simulink model "current_inverter"  (R2023a)
settings: Solver=ode4  StartTime=0.0  StopTime=0.8  FixedStep=1e-6  RelTol=1e-3
undefined symbols (not defined in the file): omega, vref_rms
libraries: spsThreePhaseVIMeasurementLib x5, spsHalfBridgeConverterLib x3, spsGroundLib x2, eeGeneralControl x2, spsPower3phInstantaneousLib x2, spsThreePhaseSeriesRLCBranchLib x2, spsAlphaBetaZerotoabcLib x1, spsDCVoltageSourceLib x1, spsPLL3phLib x1, spsRMSLib x1, eePwmGeneratorTwoLevel x1, spsThreePhaseParallelRLCBranchLib x1
settings Model: Creator=MrSam  LastModifiedBy=15185

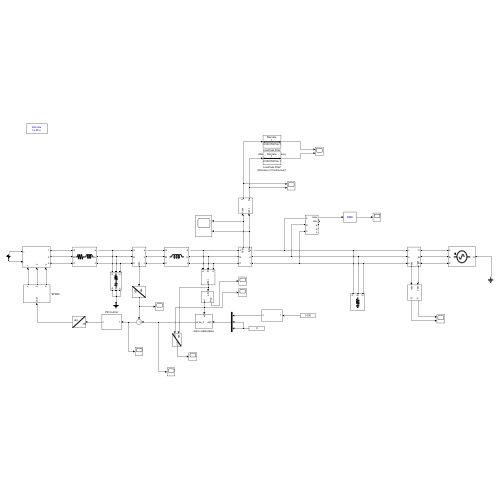
[thumbnail: Simulink's stored preview of the top-level diagram]
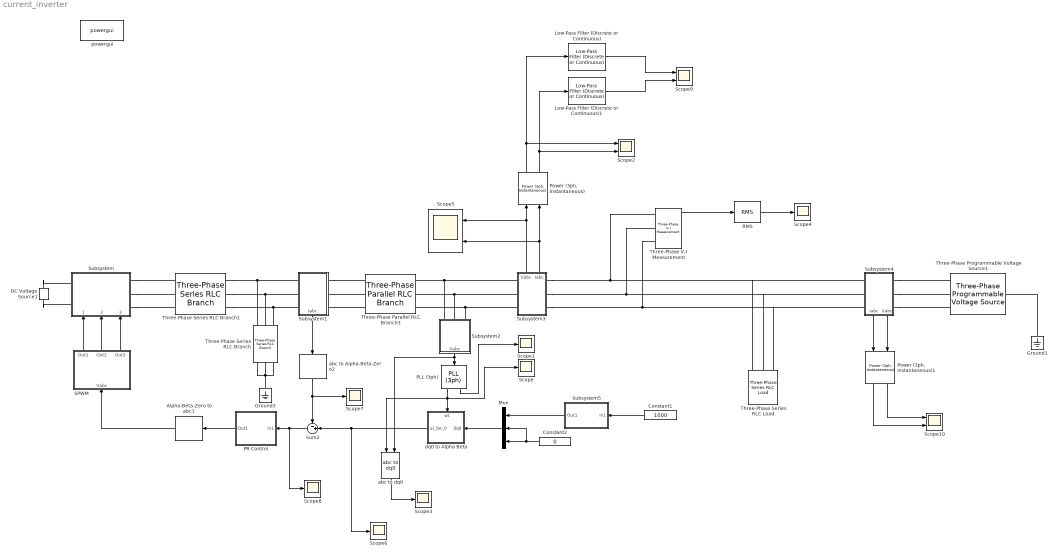
== system current_inverter ==
  Alpha-Beta-Zero to abc1 : spsAlphaBetaZerotoabcLib/Alpha-Beta-Zero to abc
      settings: LibrarySourceBlock=|
      | sps_lib/Control/Alpha-Beta-Zero
      | to abc
  Constant1 : Constant  Value=1000
  Constant2 : Constant  Value=0
  DC Voltage Source1 : spsDCVoltageSourceLib/DC Voltage Source  Amplitude=600  Measurements=None
  Ground1 : spsGroundLib/Ground  LConnTagsString=a
  Ground3 : spsGroundLib/Ground  LConnTagsString=a
  Low-Pass Filter (Discrete or Continuous) : eeGeneralControl/Low-Pass Filter (Discrete or Continuous)  K=1  T=1/(2*pi*1000)  B=inf  A=-inf  init_option=Inherited from block input  x0=0  Ts=-1
  Low-Pass Filter (Discrete or Continuous)1 : eeGeneralControl/Low-Pass Filter (Discrete or Continuous)  K=1  T=1/(2*pi*1000)  B=inf  A=-inf  init_option=Inherited from block input  x0=0  Ts=-1
  Mux : Mux  Inputs=3
  PLL (3ph) : spsPLL3phLib/PLL (3ph)  Fmin=45  Par_Init=[0, 50]  ParK=[180, 3200, 1]  TcD=1e-4  MaxRateChangeFreq=12  FilterCutOffFreq=25  Ts=0  AGC=on
  PR Control : Subsystem
  "Power (3ph, Instantaneous)" : spsPower3phInstantaneousLib/Power (3ph, Instantaneous)
  "Power (3ph, Instantaneous)1" : spsPower3phInstantaneousLib/Power (3ph, Instantaneous)
  RMS : spsRMSLib/RMS  TrueRMS=on  Freq=50  RMSInit=120  Ts=0
  SPWM : Subsystem
  Scope{,1,3..4,6..8} (7 alike) : Scope
  Scope{2,5,9..10} (4 alike) : Scope  NumInputPorts=2
  Subsystem : Subsystem
      settings: PortSchema="{\"entries\":[{\"content\":{\"sides\":[{\"content\":{\"connectorIds\":[\"LConn1\",\"LConn2\"]},\"type\":\"ConnectorPlacement.EquallySpacedRectSide\",\"uuid\":\"21765539-0567-4900-b052-fb0c809e49e6\"},{\"content\":{\"connectorIds\":[\"RConn1\",\"RConn2\",\"RConn3\"],\"side\":\"RIGHT\"},\"type\":\"ConnectorPlacement.EquallySpacedRectSide\",\"uuid\":\"da60e673-aefd-4ef6-b5b1-e42a137712f7\"},{\"content\":{\"side\":\"TOP\"},\"type\":\"ConnectorPlacement.EquallySpacedRectSide\",\"uuid\":\"b6e664be-1a8c-4c9c-bd73-b93bd6e53381\"},{\"content\":{\"connectorIds\":[\"In1\",\"In2\",\"In3\"],\"side\":\"BOTTOM\"},\"type\":\"ConnectorPlacement.EquallySpacedRectSide\",\"uuid\":\"f785bed7-33ce-41e0-9620-ddd9724794f7\"}]},\"type\":\"ConnectorPlacement.EquallySpacedConnector\",\"uuid\":\"3eaff965-cae1-44ee-8f3f-ae8df46f200b\"}],\"packageUris\":[\"http://schema.mathworks.com/mf0/Connector/R2020b\"],\"version\":\"1.0\"}"
  Subsystem1 : Subsystem
      settings: PortSchema="{\"entries\":[{\"content\":{\"sides\":[{\"content\":{\"connectorIds\":[\"LConn1\",\"LConn2\",\"LConn3\"]},\"type\":\"ConnectorPlacement.EquallySpacedRectSide\",\"uuid\":\"5e649b81-8d67-47fb-b51d-7fa1d294a0fa\"},{\"content\":{\"connectorIds\":[\"RConn1\",\"RConn2\",\"RConn3\"],\"side\":\"RIGHT\"},\"type\":\"ConnectorPlacement.EquallySpacedRectSide\",\"uuid\":\"b8ce6232-1e24-4620-bb1d-7a04b9b53c9d\"},{\"content\":{\"side\":\"TOP\"},\"type\":\"ConnectorPlacement.EquallySpacedRectSide\",\"uuid\":\"aabe5581-fbc6-4714-8701-49215a0525de\"},{\"content\":{\"connectorIds\":[\"Out1\"],\"side\":\"BOTTOM\"},\"type\":\"ConnectorPlacement.EquallySpacedRectSide\",\"uuid\":\"d004e6ed-4fae-491a-82a2-0495bcb0f8c1\"}]},\"type\":\"ConnectorPlacement.EquallySpacedConnector\",\"uuid\":\"9c494b08-2ee2-4375-b64d-9899f5cce3ba\"}],\"packageUris\":[\"http://schema.mathworks.com/mf0/Connector/R2020b\"],\"version\":\"1.0\"}"
  Subsystem2 : Subsystem
  Subsystem3 : Subsystem
      settings: PortSchema="{\"entries\":[{\"content\":{\"sides\":[{\"content\":{\"connectorIds\":[\"LConn1\",\"LConn2\",\"LConn3\"]},\"type\":\"ConnectorPlacement.EquallySpacedRectSide\",\"uuid\":\"5e649b81-8d67-47fb-b51d-7fa1d294a0fa\"},{\"content\":{\"connectorIds\":[\"RConn1\",\"RConn2\",\"RConn3\"],\"side\":\"RIGHT\"},\"type\":\"ConnectorPlacement.EquallySpacedRectSide\",\"uuid\":\"b8ce6232-1e24-4620-bb1d-7a04b9b53c9d\"},{\"content\":{\"connectorIds\":[\"Out1\",\"Out2\"],\"side\":\"TOP\"},\"type\":\"ConnectorPlacement.EquallySpacedRectSide\",\"uuid\":\"aabe5581-fbc6-4714-8701-49215a0525de\"}]},\"type\":\"ConnectorPlacement.EquallySpacedConnector\",\"uuid\":\"9c494b08-2ee2-4375-b64d-9899f5cce3ba\"}],\"packageUris\":[\"http://schema.mathworks.com/mf0/Connector/R2020b\"],\"version\":\"1.0\"}"
  Subsystem4 : Subsystem
      settings: PortSchema="{\"entries\":[{\"content\":{\"sides\":[{\"content\":{\"connectorIds\":[\"LConn1\",\"LConn2\",\"LConn3\"]},\"type\":\"ConnectorPlacement.EquallySpacedRectSide\",\"uuid\":\"5e649b81-8d67-47fb-b51d-7fa1d294a0fa\"},{\"content\":{\"connectorIds\":[\"RConn1\",\"RConn2\",\"RConn3\"],\"side\":\"RIGHT\"},\"type\":\"ConnectorPlacement.EquallySpacedRectSide\",\"uuid\":\"b8ce6232-1e24-4620-bb1d-7a04b9b53c9d\"},{\"content\":{\"connectorIds\":[\"Out1\",\"Out2\"],\"side\":\"TOP\"},\"type\":\"ConnectorPlacement.EquallySpacedRectSide\",\"uuid\":\"aabe5581-fbc6-4714-8701-49215a0525de\"}]},\"type\":\"ConnectorPlacement.EquallySpacedConnector\",\"uuid\":\"9c494b08-2ee2-4375-b64d-9899f5cce3ba\"}],\"packageUris\":[\"http://schema.mathworks.com/mf0/Connector/R2020b\"],\"version\":\"1.0\"}"
  Subsystem5 : Subsystem
  Sum2 : Sum  Inputs=-+|
  Three-Phase Parallel RLC Branch3 : spsThreePhaseParallelRLCBranchLib/Three-Phase Parallel RLC Branch  LConnTagsString=A|B|C  RConnTagsString=A|B|C  BranchType=L  Resistance=1  Inductance=0.00024  Capacitance=1e-6  Measurements=None
  Three-Phase Programmable Voltage Source1 : spsThreePhaseProgrammableVoltageSourceLib/Three-Phase Programmable Voltage Source  PositiveSequence="[vref_rms  0 50]"  VariationEntity=None  VariationType=Table of time-amplitude pairs  VariationTypeAlt=Step  VariationStep=0.5  VariationRate=10  VariationMagnitude=0.3  VariationFrequency=2  VariationTiming=[1 2]  VariationPhaseA=off  Amplitudes=[1 0.8 1.2 1.0]  TimeValues=[0 0.1 0.15 0.2]  HarmonicGeneration=off  HarmonicA=[3 0.2 -25 0]  HarmonicB=[2 0.15 35 2]  Timing="[0.05  3]"  BusType=swing  Pref=0  Qref=0  Qmin=-inf  Qmax=inf
  Three-Phase Series RLC Branch : spsThreePhaseSeriesRLCBranchLib/Three-Phase Series RLC Branch  LConnTagsString=A|B|C  RConnTagsString=A|B|C  BranchType=RC  Resistance=1  Inductance=1e-3  Capacitance=2e-05  Measurements=None
  Three-Phase Series RLC Branch1 : spsThreePhaseSeriesRLCBranchLib/Three-Phase Series RLC Branch  LConnTagsString=A|B|C  RConnTagsString=A|B|C  BranchType=RL  Resistance=0.3  Inductance=0.004  Capacitance=1e-6  Measurements=None
  Three-Phase Series RLC Load : spsThreePhaseSeriesRLCLoadLib/Three-Phase Series RLC Load  LConnTagsString=A|B|C  Configuration=Y (grounded)  NominalVoltage=367  Vabc=[1e3 1e3 1e3]  Vabcp=[1e3 1e3 1e3]  NominalFrequency=50  UnbalancedPower=off  ActivePower=1000  InductivePower=0  CapacitivePower=0  Pabc=[10e3 9e3 11e3]  QLabc=[100 90 110]  QCabc=[100 90 110]  Pabcp=[10e3 9e3 11e3]  QLabcp=[100 90 110]  QCabcp=[100 90 110]  Measurements=None  LoadType=constant Z
  Three-Phase V-I Measurement : spsThreePhaseVIMeasurementLib/Three-Phase V-I Measurement  VoltageMeasurement=phase-to-phase  SetLabelV=off  LabelV=Vabc  Vpu=off  VpuLL=off  CurrentMeasurement=yes  SetLabelI=off  LabelI=Iabc  Ipu=off  Pbase=100e6  Vbase=500e3  OutputType=Complex  PhasorSimulation=off  PSBequivalent=0
  abc to Alpha-Beta-Zero2 : spsabctoAlphaBetaZeroLib/abc to Alpha-Beta-Zero
  abc to dq0 : spsabctodq0Lib/abc to dq0  Alignment=90 degrees behind phase A axis
  dq0 to Alpha Beta : Subsystem
      settings: PortSchema="{\"entries\":[{\"content\":{\"sides\":[{\"content\":{\"connectorIds\":[\"In1\"]},\"type\":\"ConnectorPlacement.EquallySpacedRectSide\",\"uuid\":\"2957cf7a-c1c3-4848-9407-b6952c647f30\"},{\"content\":{\"connectorIds\":[\"Out1\"],\"side\":\"RIGHT\"},\"type\":\"ConnectorPlacement.EquallySpacedRectSide\",\"uuid\":\"7a8beffb-254d-479d-a697-96ba44ae1442\"},{\"content\":{\"connectorIds\":[\"In2\"],\"side\":\"TOP\"},\"type\":\"ConnectorPlacement.EquallySpacedRectSide\",\"uuid\":\"8b95608f-2c8d-45bf-9e71-a12dce74a0a0\"}]},\"type\":\"ConnectorPlacement.EquallySpacedConnector\",\"uuid\":\"69f38502-e33d-4dbf-872c-0372c4b36551\"}],\"packageUris\":[\"http://schema.mathworks.com/mf0/Connector/R2020b\"],\"version\":\"1.0\"}"
  powergui : spspowerguiLib/powergui  Priority=1  SimulationMode=Discrete  SampleTime=1e-6  frequency=60  Iterations=50  frequencyindice=50  Pbase=100e6  ErrMax=1e-4  UnitsV=kV  UnitsW=MW  buscounter=0  FunctionMessages=off  echomessages=off  EnableUseOfTLC=off  CurrentSourceSwitches=off  DisableSnubberDevices=off  DisableRonSwitches=off  DisableVfSwitches=off  DisplayEquations=off  AutomaticDiscreteSolvers=off  SolverType=Tustin/Backward Euler (TBE)  Interpol=off  ExternalGateDelay=off  methode=off  Ts=100  x0status=blocks  SPID=on  SwTol=0  HookPort=off  NonlinearTolerance=1e-4  nMaxIteration=100  ContinueOnMaxIteration=off  RestoreLinks=warning  ResistiveCurrentMeasurement=off  Frange=[0:2:500]  Ylog=off  Xlog=on  ShowGrid=off  save=off  variable=ZData  structure=0  ZoomFFT=off  StartTime=0.0  cycles=1  DisplayStyle=1  fundamental=60  FreqAxis=off  MaxFrequency=1000  frequencyindicesteady=1  RmsSteady=1  display=off
  wires:
  SPWM/1(Out1) -> Subsystem/1(" 1 ")
  SPWM/2(Out2) -> Subsystem/2("  2")
  SPWM/3(Out3) -> Subsystem/3("  3")
  Subsystem1/1(Iabc) -> abc to Alpha-Beta-Zero2/1
  Subsystem3/2(Iabc) -> Scope5/2, "Power (3ph, Instantaneous)"/2
  Subsystem3/1(Vabc) -> "Power (3ph, Instantaneous)"/1, Scope5/1
  Sum2/1 -> Scope8/1, PR Control/1(In1)
  PR Control/1(Out1) -> Alpha-Beta-Zero to abc1/1
  Subsystem2/1(Vabc) -> abc to dq0/1, PLL (3ph)/1
  dq0 to Alpha Beta/1(al_be_0) -> Scope6/1, Sum2/2
  Mux/1 -> dq0 to Alpha Beta/1(dq0)
  PLL (3ph)/2 -> abc to dq0/2, dq0 to Alpha Beta/2(wt), Scope/1
  Constant2/1 -> Mux/2, Mux/3
  PLL (3ph)/1 -> Scope1/1
  "Power (3ph, Instantaneous)"/1 -> Low-Pass Filter (Discrete or Continuous)/1, Scope2/1
  "Power (3ph, Instantaneous)"/2 -> Low-Pass Filter (Discrete or Continuous)1/1, Scope2/2
  abc to dq0/1 -> Scope3/1
  Alpha-Beta-Zero to abc1/1 -> SPWM/1(Vabc)
  abc to Alpha-Beta-Zero2/1 -> Scope7/1, Sum2/1
  Low-Pass Filter (Discrete or Continuous)/1 -> Scope9/1
  Low-Pass Filter (Discrete or Continuous)1/1 -> Scope9/2
  Three-Phase V-I Measurement/1 -> RMS/1
  RMS/1 -> Scope4/1
  Subsystem4/2(Iabc) -> "Power (3ph, Instantaneous)1"/2
  Subsystem4/1(Vabc) -> "Power (3ph, Instantaneous)1"/1
  "Power (3ph, Instantaneous)1"/1 -> Scope10/1
  "Power (3ph, Instantaneous)1"/2 -> Scope10/2
  Subsystem5/1(Out1) -> Mux/1
  Constant1/1 -> Subsystem5/1(In1)
  connections:
  Ground3/LConn1 -- Three-Phase Series RLC Branch/RConn3 -- Three-Phase Series RLC Branch/RConn1 -- Three-Phase Series RLC Branch/RConn2
  DC Voltage Source1/RConn1 -- Subsystem/LConn1
  DC Voltage Source1/LConn1 -- Subsystem/LConn2
  Three-Phase Series RLC Branch/LConn1 -- Three-Phase Series RLC Branch1/RConn1 -- Subsystem1/LConn1
  Three-Phase Series RLC Branch/LConn2 -- Three-Phase Series RLC Branch1/RConn2 -- Subsystem1/LConn2
  Three-Phase Series RLC Branch/LConn3 -- Three-Phase Series RLC Branch1/RConn3 -- Subsystem1/LConn3
  Subsystem1/RConn1 -- Three-Phase Parallel RLC Branch3/LConn1
  Subsystem1/RConn2 -- Three-Phase Parallel RLC Branch3/LConn2
  Subsystem1/RConn3 -- Three-Phase Parallel RLC Branch3/LConn3
  Subsystem2/LConn1 -- Three-Phase Parallel RLC Branch3/RConn1 -- Subsystem3/LConn1
  Subsystem2/LConn2 -- Three-Phase Parallel RLC Branch3/RConn2 -- Subsystem3/LConn2
  Subsystem2/LConn3 -- Three-Phase Parallel RLC Branch3/RConn3 -- Subsystem3/LConn3
  Subsystem3/RConn1 -- Subsystem4/RConn3 -- Three-Phase Series RLC Load/LConn1 -- Three-Phase V-I Measurement/LConn1
  Subsystem3/RConn2 -- Subsystem4/RConn2 -- Three-Phase Series RLC Load/LConn2 -- Three-Phase V-I Measurement/LConn2
  Subsystem3/RConn3 -- Subsystem4/RConn1 -- Three-Phase Series RLC Load/LConn3 -- Three-Phase V-I Measurement/LConn3
  Ground1/LConn1 -- Three-Phase Programmable Voltage Source1/LConn1
  Subsystem/RConn2 -- Three-Phase Series RLC Branch1/LConn2
  Subsystem/RConn1 -- Three-Phase Series RLC Branch1/LConn1
  Subsystem/RConn3 -- Three-Phase Series RLC Branch1/LConn3
  Subsystem4/LConn3 -- Three-Phase Programmable Voltage Source1/RConn1
  Subsystem4/LConn2 -- Three-Phase Programmable Voltage Source1/RConn2
  Subsystem4/LConn1 -- Three-Phase Programmable Voltage Source1/RConn3

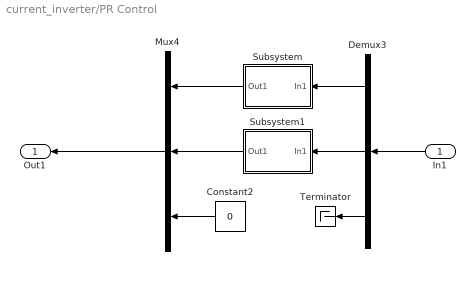
== system current_inverter/PR Control ==
  In1 : Inport
  Constant2 : Constant  Value=0
  Demux3 : Demux  Outputs=3
  Mux4 : Mux  Inputs=3
  Subsystem : Subsystem
  Subsystem1 : Subsystem
  Terminator : Terminator
  Out1 : Outport
  wires:
  Mux4/1 -> Out1/1
  Constant2/1 -> Mux4/3
  In1/1 -> Demux3/1
  Demux3/3 -> Terminator/1
  Demux3/1 -> Subsystem/1(In1)
  Subsystem/1(Out1) -> Mux4/1
  Subsystem1/1(Out1) -> Mux4/2
  Demux3/2 -> Subsystem1/1(In1)

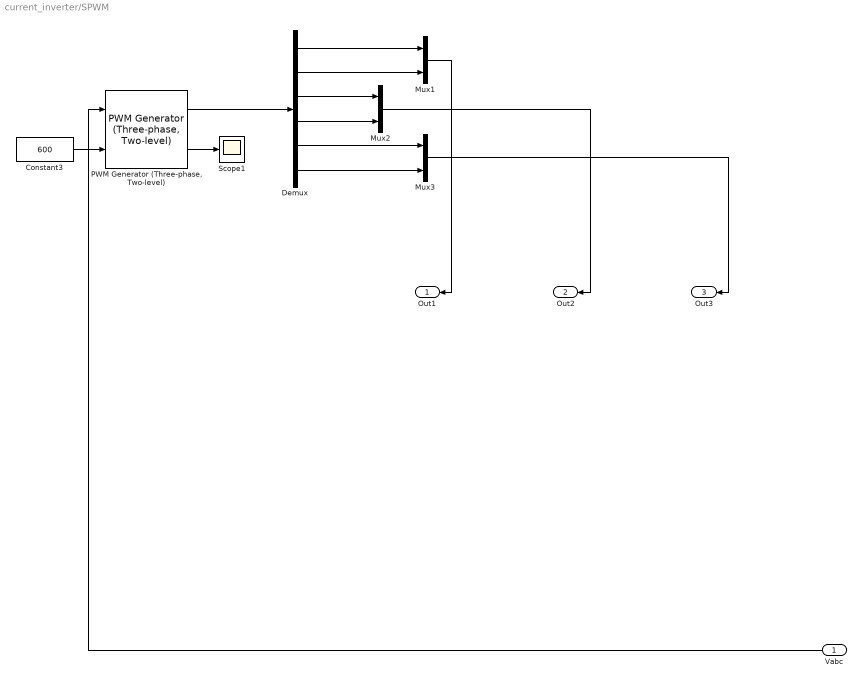
== system current_inverter/SPWM ==
  Vabc : Inport
  Constant3 : Constant  Value=600
  Demux : Demux  Outputs=6
  Mux1 : Mux  Inputs=2
  Mux2 : Mux  Inputs=2
  Mux3 : Mux  Inputs=2
  "PWM Generator (Three-phase, Two-level)" : eePwmGeneratorTwoLevel/PWM Generator (Three-phase, Two-level)  PWMMode=Continuous PWM (CPWM)  CPWMMode=SPWM: sinusoidal PWM  DPWMMode=60 DPWM: 60 degree discontinuous PWM  fsw=10000  Ts=1/(100*10000)
      settings: LibrarySourceBlock=|
      | ee_sl_lib/Pulse Width
      | Modulation/PWM Generator
      | (Three-phase, Two-level)
  Scope1 : Scope
  Out1 : Outport
  Out2 : Outport  Port=2
  Out3 : Outport  Port=3
  wires:
  "PWM Generator (Three-phase, Two-level)"/2 -> Scope1/1
  Demux/2 -> Mux1/2
  Vabc/1 -> "PWM Generator (Three-phase, Two-level)"/1
  Demux/6 -> Mux3/2
  Demux/1 -> Mux1/1
  Constant3/1 -> "PWM Generator (Three-phase, Two-level)"/2
  Mux2/1 -> Out2/1
  Demux/4 -> Mux2/2
  "PWM Generator (Three-phase, Two-level)"/1 -> Demux/1
  Demux/3 -> Mux2/1
  Demux/5 -> Mux3/1
  Mux1/1 -> Out1/1
  Mux3/1 -> Out3/1

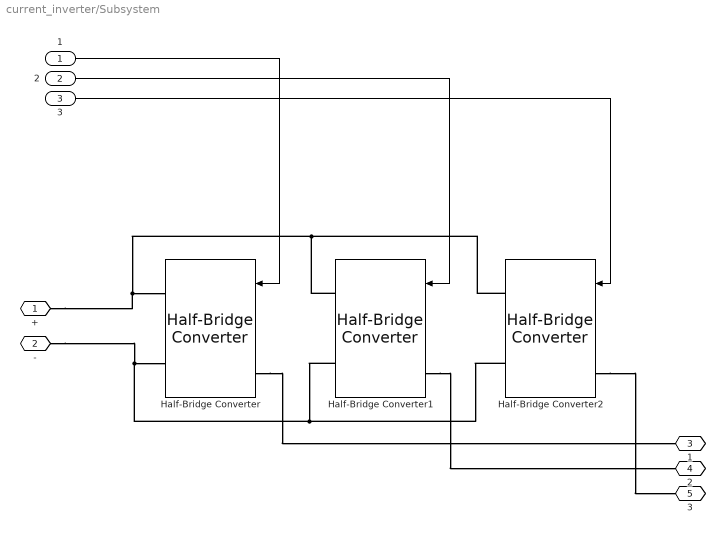
== system current_inverter/Subsystem ==
  " 1 " : Inport
  "  2" : Inport  Port=2
  "  3" : Inport  Port=3
  Half-Bridge Converter : spsHalfBridgeConverterLib/Half-Bridge Converter  ModelType=Switching devices  Ron=1e-3  Rs=1e6  Cs=inf  Vforward=[0,0]  Ron_Diode=1e-3  Rs_Diode=1e6  Cs_Diode=inf  Vf_Diode=1e-3  Rs_CurrentSource=inf  Ron_ACsource=1e-3
      settings: LibrarySourceBlock=sps_lib/Power Electronics/Half-Bridge Converter
  Half-Bridge Converter1 : spsHalfBridgeConverterLib/Half-Bridge Converter  ModelType=Switching devices  Ron=1e-3  Rs=1e6  Cs=inf  Vforward=[0,0]  Ron_Diode=1e-3  Rs_Diode=1e6  Cs_Diode=inf  Vf_Diode=1e-3  Rs_CurrentSource=inf  Ron_ACsource=1e-3
      settings: LibrarySourceBlock=sps_lib/Power Electronics/Half-Bridge Converter
  Half-Bridge Converter2 : spsHalfBridgeConverterLib/Half-Bridge Converter  ModelType=Switching devices  Ron=1e-3  Rs=1e6  Cs=inf  Vforward=[0,0]  Ron_Diode=1e-3  Rs_Diode=1e6  Cs_Diode=inf  Vf_Diode=1e-3  Rs_CurrentSource=inf  Ron_ACsource=1e-3
      settings: LibrarySourceBlock=sps_lib/Power Electronics/Half-Bridge Converter
  + : PMIOPort  Side=Left
  - : PMIOPort  Port=2  Side=Left
  1 : PMIOPort  Port=3  Side=Right
  2 : PMIOPort  Port=4  Side=Right
  3 : PMIOPort  Port=5  Side=Right
  wires:
  "  2"/1 -> Half-Bridge Converter1/1
  "  3"/1 -> Half-Bridge Converter2/1
  " 1 "/1 -> Half-Bridge Converter/1
  connections:
  Half-Bridge Converter/LConn1 -- 1/RConn1
  Half-Bridge Converter2/RConn1 -- Half-Bridge Converter1/RConn1 -- Half-Bridge Converter/RConn1 -- +/RConn1
  Half-Bridge Converter2/RConn2 -- Half-Bridge Converter1/RConn2 -- Half-Bridge Converter/RConn2 -- -/RConn1
  Half-Bridge Converter2/LConn1 -- 3/RConn1
  Half-Bridge Converter1/LConn1 -- 2/RConn1

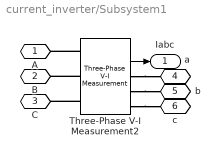
== system current_inverter/Subsystem1 ==
  Three-Phase V-I Measurement2 : spsThreePhaseVIMeasurementLib/Three-Phase V-I Measurement  VoltageMeasurement=phase-to-ground  SetLabelV=off  LabelV=Vabc  Vpu=off  VpuLL=off  CurrentMeasurement=yes  SetLabelI=off  LabelI=Iabc  Ipu=off  Pbase=100e6  Vbase=500e3  OutputType=Complex  PhasorSimulation=off  PSBequivalent=0
  A : PMIOPort  Side=Left
  B : PMIOPort  Port=2  Side=Left
  C : PMIOPort  Port=3  Side=Left
  a : PMIOPort  Port=4  Side=Right
  b : PMIOPort  Port=5  Side=Right
  c : PMIOPort  Port=6  Side=Right
  Iabc : Outport
  wires:
  Three-Phase V-I Measurement2/2 -> Iabc/1
  connections:
  Three-Phase V-I Measurement2/LConn1 -- A/RConn1
  Three-Phase V-I Measurement2/RConn3 -- c/RConn1
  Three-Phase V-I Measurement2/RConn1 -- a/RConn1
  Three-Phase V-I Measurement2/LConn2 -- B/RConn1
  Three-Phase V-I Measurement2/RConn2 -- b/RConn1
  Three-Phase V-I Measurement2/LConn3 -- C/RConn1

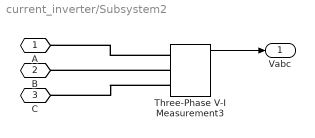
== system current_inverter/Subsystem2 ==
  Three-Phase V-I Measurement3 : spsThreePhaseVIMeasurementLib/Three-Phase V-I Measurement  VoltageMeasurement=phase-to-ground  SetLabelV=off  LabelV=Vabc  Vpu=off  VpuLL=off  CurrentMeasurement=yes  SetLabelI=off  LabelI=Iabc  Ipu=off  Pbase=100e6  Vbase=500e3  OutputType=Complex  PhasorSimulation=off  PSBequivalent=0
  A : PMIOPort  Side=Left
  B : PMIOPort  Port=2  Side=Left
  C : PMIOPort  Port=3  Side=Left
  Vabc : Outport
  wires:
  Three-Phase V-I Measurement3/1 -> Vabc/1
  connections:
  Three-Phase V-I Measurement3/LConn1 -- A/RConn1
  Three-Phase V-I Measurement3/LConn2 -- B/RConn1
  Three-Phase V-I Measurement3/LConn3 -- C/RConn1

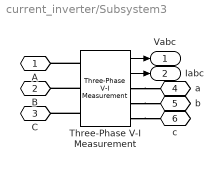
== system current_inverter/Subsystem3 ==
  Three-Phase V-I Measurement : spsThreePhaseVIMeasurementLib/Three-Phase V-I Measurement  VoltageMeasurement=phase-to-ground  SetLabelV=off  LabelV=Vabc  Vpu=off  VpuLL=off  CurrentMeasurement=yes  SetLabelI=off  LabelI=Iabc  Ipu=off  Pbase=100e6  Vbase=500e3  OutputType=Complex  PhasorSimulation=off  PSBequivalent=0
  A : PMIOPort  Side=Left
  B : PMIOPort  Port=2  Side=Left
  C : PMIOPort  Port=3  Side=Left
  a : PMIOPort  Port=4  Side=Right
  b : PMIOPort  Port=5  Side=Right
  c : PMIOPort  Port=6  Side=Right
  Vabc : Outport
  Iabc : Outport  Port=2
  wires:
  Three-Phase V-I Measurement/2 -> Iabc/1
  Three-Phase V-I Measurement/1 -> Vabc/1
  connections:
  Three-Phase V-I Measurement/RConn1 -- a/RConn1
  Three-Phase V-I Measurement/LConn2 -- B/RConn1
  Three-Phase V-I Measurement/RConn3 -- c/RConn1
  Three-Phase V-I Measurement/LConn1 -- A/RConn1
  Three-Phase V-I Measurement/LConn3 -- C/RConn1
  Three-Phase V-I Measurement/RConn2 -- b/RConn1

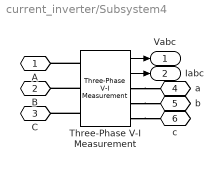
== system current_inverter/Subsystem4 ==
  Three-Phase V-I Measurement : spsThreePhaseVIMeasurementLib/Three-Phase V-I Measurement  VoltageMeasurement=phase-to-ground  SetLabelV=off  LabelV=Vabc  Vpu=off  VpuLL=off  CurrentMeasurement=yes  SetLabelI=off  LabelI=Iabc  Ipu=off  Pbase=100e6  Vbase=500e3  OutputType=Complex  PhasorSimulation=off  PSBequivalent=0
  A : PMIOPort  Side=Left
  B : PMIOPort  Port=2  Side=Left
  C : PMIOPort  Port=3  Side=Left
  a : PMIOPort  Port=4  Side=Right
  b : PMIOPort  Port=5  Side=Right
  c : PMIOPort  Port=6  Side=Right
  Vabc : Outport
  Iabc : Outport  Port=2
  wires:
  Three-Phase V-I Measurement/2 -> Iabc/1
  Three-Phase V-I Measurement/1 -> Vabc/1
  connections:
  Three-Phase V-I Measurement/RConn1 -- a/RConn1
  Three-Phase V-I Measurement/LConn2 -- B/RConn1
  Three-Phase V-I Measurement/RConn3 -- c/RConn1
  Three-Phase V-I Measurement/LConn1 -- A/RConn1
  Three-Phase V-I Measurement/LConn3 -- C/RConn1
  Three-Phase V-I Measurement/RConn2 -- b/RConn1

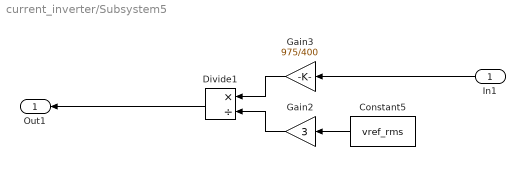
== system current_inverter/Subsystem5 ==
  In1 : Inport
  Constant5 : Constant  Value=vref_rms
  Divide1 : Product  Inputs=*/
  Gain2 : Gain  Gain=3
  Gain3 : Gain  Gain=975/400
  Out1 : Outport
  wires:
  Gain3/1 -> Divide1/1
  Constant5/1 -> Gain2/1
  Gain2/1 -> Divide1/2
  In1/1 -> Gain3/1
  Divide1/1 -> Out1/1

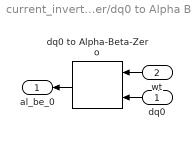
== system current_inverter/dq0 to Alpha Beta ==
  dq0 : Inport
  wt : Inport  Port=2
  dq0 to Alpha-Beta-Zero : spsdq0toAlphaBetaZeroLib/dq0 to Alpha-Beta-Zero  Alignment=90 degrees behind phase A axis
  al_be_0 : Outport
  wires:
  dq0 to Alpha-Beta-Zero/1 -> al_be_0/1
  wt/1 -> dq0 to Alpha-Beta-Zero/2
  dq0/1 -> dq0 to Alpha-Beta-Zero/1

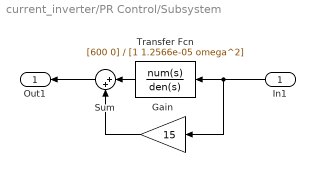
== system current_inverter/PR Control/Subsystem ==
  In1 : Inport
  Gain : Gain  Gain=15
  Sum : Sum  Inputs=|++
  Transfer Fcn : TransferFcn  Numerator=[600 0]  Denominator=[1 1.2566e-05 omega^2]
  Out1 : Outport
  wires:
  Sum/1 -> Out1/1
  In1/1 -> Transfer Fcn/1, Gain/1
  Transfer Fcn/1 -> Sum/1
  Gain/1 -> Sum/2

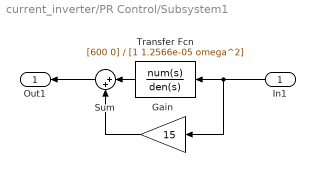
== system current_inverter/PR Control/Subsystem1 ==
  In1 : Inport
  Gain : Gain  Gain=15
  Sum : Sum  Inputs=|++
  Transfer Fcn : TransferFcn  Numerator=[600 0]  Denominator=[1 1.2566e-05 omega^2]
  Out1 : Outport
  wires:
  Sum/1 -> Out1/1
  In1/1 -> Transfer Fcn/1, Gain/1
  Transfer Fcn/1 -> Sum/1
  Gain/1 -> Sum/2
